simulink model "MyEngine_RTW"  (Simulink 7.5)
settings: Solver=ode1  SolverMode=SingleTasking  StartTime=0.0  StopTime=inf  FixedStep=0.0002  RelTol=1e-3
PreLoadFcn:
  | vehicle = 'Car'; if ~length(which('cmcmd')), cmenv; end
  | MyEngine_RTW_bus
InitFcn:
  | vehicle = 'Car'; if ~length(which('cmcmd')), cmenv; end
  | MyEngine_RTW_bus
libraries: simulink x2, CarMaker4SL x2
Description:
  | CarMaker Real-Time Target (generic)
settings Model: Creator=ml  LastModifiedBy=ml
settings DebuggingCC: SolverPrmCheckMsg=none
settings HardwareCC: TargetHWDeviceType=32-bit Generic  ProdEqTarget=off
settings RTWCC: SystemTargetFile=CarMaker.tlc  TemplateMakefile=CarMaker_unix.tmf  Description=CarMaker Real-Time Target (32-bit)  ProcessScript=CarMaker_make_rtw_hook
settings CodeAppCC: MaxIdLength=63
settings STFCustomTargetCC: ModelReferenceCompliant=off  GeneratePreprocessorConditionals=Disable all  SystemTargetFile=CarMaker.tlc
settings GRTTargetCC: ModelReferenceCompliant=off  ParMdlRefBuildCompliant=off  CompOptLevelCompliant=off  MatFileLogging=off  ExtModeMexFile=noextcomm
settings CustomProperty: DataType=string  Value=..
settings EnumStrPairs: String=Car

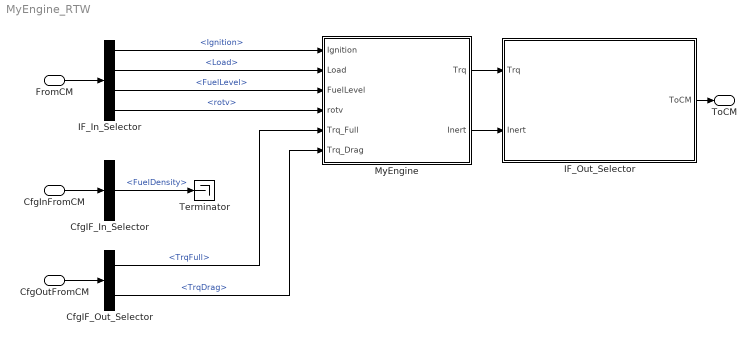
== system MyEngine_RTW ==
  FromCM : Inport  UseBusObject=on
      settings: BusObject=cmPTEngineIn
  CfgInFromCM : Inport  Port=2  UseBusObject=on
      settings: BusObject=cmPTEngineCfgIn
  CfgOutFromCM : Inport  Port=3  UseBusObject=on
      settings: BusObject=cmPTEngineCfgOut
  CfgIF_In_Selector : BusSelector  OutputSignals=FuelDensity
  CfgIF_Out_Selector : BusSelector  OutputSignals=TrqFull,TrqDrag
  IF_In_Selector : BusSelector  OutputSignals=Ignition,Load,FuelLevel,rotv
  IF_Out_Selector : Subsystem
      settings: OpenFcn=cmSignalSelect('SignalSelection_CB',gcb)
      mask Type: Signal Selection
      mask Description: Signal Selection Block
  MyEngine : Subsystem
  Terminator : Terminator
  ToCM : Outport  UseBusObject=on
      settings: BusObject=cmPTEngineOut
  wires:
  FromCM/1 -> IF_In_Selector/1
  IF_Out_Selector/1(ToCM) -> ToCM/1
  CfgInFromCM/1 -> CfgIF_In_Selector/1
  CfgOutFromCM/1 -> CfgIF_Out_Selector/1
  IF_In_Selector/1 -> MyEngine/1(Ignition)  "<Ignition>"
  IF_In_Selector/2 -> MyEngine/2(Load)  "<Load>"
  IF_In_Selector/3 -> MyEngine/3(FuelLevel)  "<FuelLevel>"
  IF_In_Selector/4 -> MyEngine/4(rotv)  "<rotv>"
  CfgIF_Out_Selector/1 -> MyEngine/5(Trq_Full)  "<TrqFull>"
  CfgIF_Out_Selector/2 -> MyEngine/6(Trq_Drag)  "<TrqDrag>"
  MyEngine/2(Inert) -> IF_Out_Selector/2(Inert)
  MyEngine/1(Trq) -> IF_Out_Selector/1(Trq)
  CfgIF_In_Selector/1 -> Terminator/1  "<FuelDensity>"

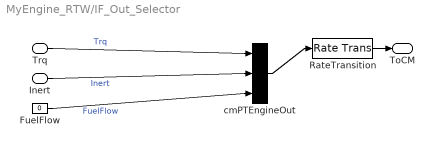
== system MyEngine_RTW/IF_Out_Selector ==
  Trq : Inport
  Inert : Inport  Port=2
  FuelFlow : Constant  Value=0
  RateTransition : RateTransition  OutPortSampleTime=str2num(get_param(gcs,'FixedStep'))
  cmPTEngineOut : BusCreator  Inputs=3
  ToCM : Outport
  wires:
  RateTransition/1 -> ToCM/1
  cmPTEngineOut/1 -> RateTransition/1
  FuelFlow/1 -> cmPTEngineOut/3  "FuelFlow"
  Trq/1 -> cmPTEngineOut/1  "Trq"
  Inert/1 -> cmPTEngineOut/2  "Inert"

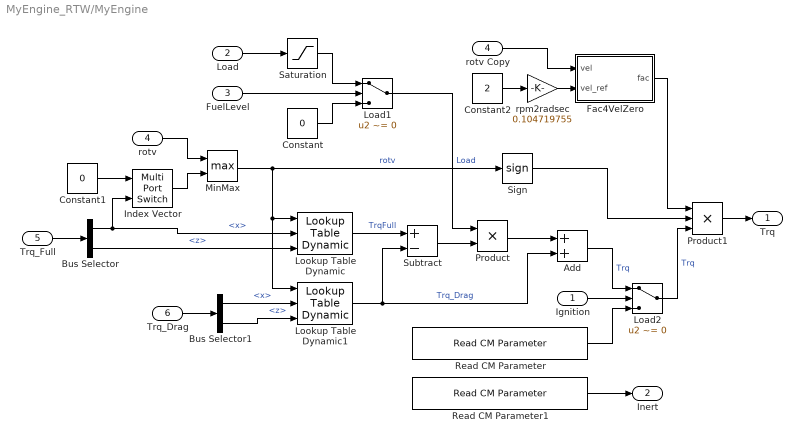
== system MyEngine_RTW/MyEngine ==
  Ignition : Inport  OutDataType=sfix(16)  OutScaling=2^0
  Load : Inport  Port=2  OutDataType=sfix(16)  OutScaling=2^0
  FuelLevel : Inport  Port=3  OutDataType=sfix(16)  OutScaling=2^0
  rotv : Inport  Port=4  OutDataType=sfix(16)  OutScaling=2^0
  Trq_Full : Inport  Port=5  OutDataType=sfix(16)  OutScaling=2^0
  Trq_Drag : Inport  Port=6  OutDataType=sfix(16)  OutScaling=2^0
  Add : Sum  OutDataType=sfix(16)  OutScaling=2^-10
  Bus Selector : BusSelector  OutputSignals=x,z
  Bus Selector1 : BusSelector  OutputSignals=x,z
  Constant : Constant  Value=0  OutDataType=sfix(16)  OutScaling=2^0
  Constant1 : Constant  Value=0  OutDataType=sfix(16)  OutScaling=2^0
  Constant2 : Constant  Value=2  OutDataType=sfix(16)  OutScaling=2^0
  Fac4VelZero : Subsystem
  Index Vector : MultiPortSwitch  DataPortOrder=Zero-based contiguous  Inputs=1  zeroidx=on  OutDataType=sfix(16)  OutScaling=2^0
  Load1 : Switch  Criteria=u2 ~= 0  OutDataType=sfix(16)  OutScaling=2^0
  Load2 : Switch  Criteria=u2 ~= 0  OutDataType=sfix(16)  OutScaling=2^0
  Lookup Table Dynamic : simulink/Lookup Tables/Lookup Table Dynamic  LookUpMeth=Interpolation-Use End Values  OutDataTypeStr=float('double')  OutputDataTypeScalingMode=Specify via dialog  OutDataType=float('double')  OutScaling=2^-10  DoSatur=off
  Lookup Table Dynamic1 : simulink/Lookup Tables/Lookup Table Dynamic  LookUpMeth=Interpolation-Use End Values  OutDataTypeStr=float('double')  OutputDataTypeScalingMode=Specify via dialog  OutDataType=float('double')  OutScaling=2^-10  DoSatur=off
  MinMax : MinMax  Function=max  Inputs=2  OutDataType=sfix(16)  OutScaling=2^0
  Product : Product  OutDataType=sfix(16)  OutScaling=2^0  RndMeth=Zero
  Product1 : Product  Inputs=3  OutDataType=sfix(16)  OutScaling=2^0  RndMeth=Zero
  Read CM Parameter : CarMaker4SL/Read CM Parameter  xfile=Vehicle  xkey=PowerTrain.MyEngine.TrqKl15Off  xnout=1  xdefaults=[]  xmuxed=on
  Read CM Parameter1 : CarMaker4SL/Read CM Parameter  xfile=Vehicle  xkey=PowerTrain.Engine.I  xnout=1  xdefaults=0.1  xmuxed=on
  Saturation : Saturate  UpperLimit=1  LowerLimit=0  OutDataType=sfix(16)  OutScaling=2^0
  Sign : Signum
  Subtract : Sum  Inputs=+-  OutDataType=sfix(16)  OutScaling=2^-10
  rotv Copy : InportShadow  Port=4  OutDataType=sfix(16)  OutScaling=2^0
  rpm2radsec : Gain  Gain=0.104719755  ParameterDataType=sfix(16)  ParameterScaling=2^0  OutDataType=sfix(16)  OutScaling=2^0
  Trq : Outport  OutDataType=sfix(16)  OutScaling=2^0
  Inert : Outport  Port=2  OutDataType=sfix(16)  OutScaling=2^0
  wires:
  Load/1 -> Saturation/1
  FuelLevel/1 -> Load1/2
  Saturation/1 -> Load1/1
  Constant/1 -> Load1/3
  Load1/1 -> Product/1  "Load"
  Ignition/1 -> Load2/2
  Read CM Parameter/1 -> Load2/3
  Read CM Parameter1/1 -> Inert/1
  Trq_Full/1 -> Bus Selector/1
  Bus Selector/1 -> Index Vector/2, Lookup Table Dynamic/2  "<x>"
  Constant1/1 -> Index Vector/1
  Index Vector/1 -> MinMax/2
  MinMax/1 -> Lookup Table Dynamic1/1, Lookup Table Dynamic/1, Sign/1  "rotv"
  Trq_Drag/1 -> Bus Selector1/1
  Bus Selector/2 -> Lookup Table Dynamic/3  "<z>"
  Bus Selector1/1 -> Lookup Table Dynamic1/2  "<x>"
  Bus Selector1/2 -> Lookup Table Dynamic1/3  "<z>"
  Lookup Table Dynamic/1 -> Subtract/1  "TrqFull"
  Lookup Table Dynamic1/1 -> Subtract/2, Add/2  "Trq_Drag"
  Subtract/1 -> Product/2
  Product/1 -> Add/1
  Add/1 -> Load2/1  "Trq"
  Product1/1 -> Trq/1
  Load2/1 -> Product1/3  "Trq"
  Constant2/1 -> rpm2radsec/1
  rpm2radsec/1 -> Fac4VelZero/2(vel_ref)
  rotv Copy/1 -> Fac4VelZero/1(vel)
  Fac4VelZero/1(fac) -> Product1/1
  Sign/1 -> Product1/2
  rotv/1 -> MinMax/1

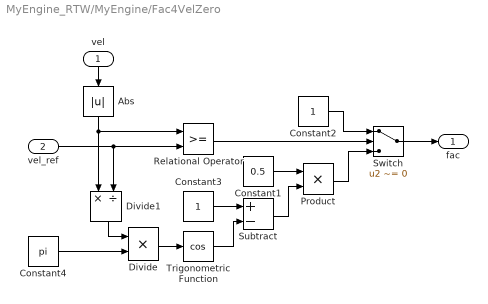
== system MyEngine_RTW/MyEngine/Fac4VelZero ==
  vel : Inport
  vel_ref : Inport  Port=2  OutDataType=sfix(16)  OutScaling=2^0
  Abs : Abs  OutDataType=sfix(16)  OutScaling=2^0
  Constant1 : Constant  Value=0.5  OutDataType=sfix(16)  OutScaling=2^0
  Constant2 : Constant  OutDataType=sfix(16)  OutScaling=2^0
  Constant3 : Constant  OutDataType=sfix(16)  OutScaling=2^0
  Constant4 : Constant  Value=pi  OutDataType=sfix(16)  OutScaling=2^0
  Divide : Product  Inputs=**  OutDataType=sfix(16)  OutScaling=2^-10
  Divide1 : Product  Inputs=*/  OutDataType=sfix(16)  OutScaling=2^-10
  Product : Product  OutDataType=sfix(16)  OutScaling=2^0  RndMeth=Zero
  Relational Operator : RelationalOperator  LogicOutDataTypeMode=boolean  OutDataTypeStr=boolean
  Subtract : Sum  Inputs=+-  OutDataType=sfix(16)  OutScaling=2^-10
  Switch : Switch  Criteria=u2 ~= 0  OutDataType=sfix(16)  OutScaling=2^0
  Trigonometric Function : Trigonometry  Operator=cos
  fac : Outport
  wires:
  Abs/1 -> Relational Operator/1, Divide1/1
  Relational Operator/1 -> Switch/2
  Constant2/1 -> Switch/1
  vel/1 -> Abs/1
  Switch/1 -> fac/1
  Product/1 -> Switch/3
  Constant1/1 -> Product/1
  Constant3/1 -> Subtract/1
  Subtract/1 -> Product/2
  Trigonometric Function/1 -> Subtract/2
  Divide/1 -> Trigonometric Function/1
  Constant4/1 -> Divide/2
  vel_ref/1 -> Relational Operator/2, Divide1/2
  Divide1/1 -> Divide/1
